simulink model "controllo_motori"  (R2025b)
settings: Solver=FixedStepAuto  StartTime=0.0  StopTime=10  FixedStep=0.01  RelTol=1e-3
libraries: slpidlib x3, vehdynlibtire x2, simulink x2, vehdynlibsteering x1, autolibshared x1
(part 2 of 2)

== matlab function controllo_motori/MATLAB Function1 ==
  data: AxlTrq input; Omega output; Vx input; Vy input; YawRate input; Omega_prev input; Fx output; Fy output; Fz output
function [Omega, Fx, Fy, Fz] = fcn(AxlTrq, Vx, Vy, YawRate, Omega_prev)
    % Parametri
    J   = 0.5;      % inerzia ruota+motore ridotta [kg·m²]
    Rw  = 0.2;      % raggio ruota [m]
    tau = 14.5;     % rapporto riduzione
    Cy  = 12000;    % rigidezza laterale pneumatico [N/rad]
    Ts  = 0.001;    % passo di integrazione [s]
    
    % Omega ruota (integrazione Eulero)
    alpha_ruota = AxlTrq / J;
    Omega = Omega_prev + alpha_ruota * Ts;
    Omega = max(0, Omega);  % no velocità negativa
    
    % Forza longitudinale
    Fx = AxlTrq * tau / Rw;
    
    % Angolo di deriva e forza laterale
    if abs(Vx) > 0.5
        slip_angle = atan2(Vy, abs(Vx)) - atan2(YawRate * 0.6, abs(Vx));
    else
        slip_angle = 0;
    end
    Fy = -Cy * slip_angle;
    
    % Forza verticale statica (peso per ruota)
    Fz = 280 * 9.81 / 4;   % [N]
end

== matlab function controllo_motori/MATLAB Function3 ==
  data: T_reqRL input; T_RL output; T_reqRR input; T_calcRL input; T_calcRR input; steerAng input; T_RR output
function [T_RL,T_RR] = fcn(T_reqRL, T_reqRR, T_calcRL, T_calcRR, steerAng)
steerAnglim = abs(3);
if abs(steerAng) < steerAnglim:
    T_RL = T_reqRL;
    T_RR = T_reqRR;
else  % in questo modo si calcola solo il delta coppia ma la coppia erogata viene scelta dal pilota
    dT = T_calcRR-T_calcRL;
    T_RL=T_reqRL-dT;
    T_RR=T_reqRR+dT;
% in questo modo si impone come coppia limite quella calcolata
    %T_RL = min(T_reqRL,T_calcRL);
    %T_RR = min(T_reqRR,T_calcRR);
